simulink model "psk_3"  (Simulink 5.1)
settings: Solver=ode45  StartTime=0.0  StopTime=2  RelTol=1e-3
values from neighbouring files (symbols this model uses):
  fc = 0.2    [TP_fdesign1.m]    (also in TP_fdesign2.m; band4.m = 2000)
  nf = 256    [band4.m]    (also in block_lms_.m = 16)
  Ts = 1/fs    (= 6.25e-05)    [G722_1.m]    (also in adaptiv_2.m = 0.001; adaptiv_3.m = 0.001; adaptiv_4.m = 0.001; adaptiv_5.m = 0.001)
undefined symbols (not defined in the file or in its folder): get, theta
libraries: dspsigops x2, dspmlti3 x2, dspsrcs4 x1, dspsnks4 x1
settings Model: Creator=svenhoffmann  LastModifiedBy=svenhoffmann  ExtModeAutoUpdateStatusClock=off  BooleanDataType=on  ProdHWDeviceType=Microprocessor

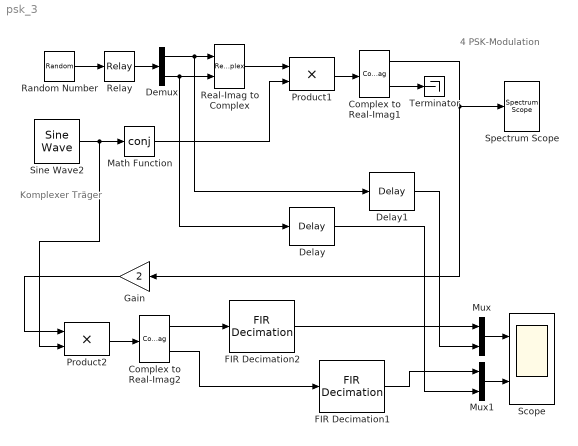
== system psk_3 ==
  note: 4 PSK-Modulation
  note: Komplexer
      | Träger
  Complex to Real-Imag1 : ComplexToRealImag
  Complex to Real-Imag2 : ComplexToRealImag
  Delay : dspsigops/Delay  dly_unit=Samples  delay=nf/2  ic_detail=off  dif_ic_for_ch=off  dif_ic_for_dly=off  ic=0  reset_popup=None
  Delay1 : dspsigops/Delay  dly_unit=Samples  delay=nf/2  ic_detail=off  dif_ic_for_ch=off  dif_ic_for_dly=off  ic=0  reset_popup=None
  Demux : Demux  Outputs=2
  FIR Decimation1 : dspmlti3/FIR Decimation  h=h0  D=10  framing=Maintain input frame size  outputBufInitCond=0  roundingMode=Floor  overflowMode=off
  FIR Decimation2 : dspmlti3/FIR Decimation  h=h0  D=10  framing=Maintain input frame size  outputBufInitCond=0  roundingMode=Floor  overflowMode=off
  Gain : Gain  Orientation=left  Gain=2  SaturateOnIntegerOverflow=on
  Math Function : Math  Operator=conj
  Mux : Mux  Inputs=2
  Mux1 : Mux  Inputs=2
  Product1 : Product  SaturateOnIntegerOverflow=on
  Product2 : Product  SaturateOnIntegerOverflow=on
  Random Number : RandomNumber  Seed=[0124, 769]  SampleTime=100*Ts
  Real-Imag to Complex : RealImagToComplex
  Relay : Relay  OffOutputValue=-1  SampleTime=Ts
  Scope : Scope  NumInputPorts=2
      settings: YMin=-1.5~-1.5  YMax=1.5~1.5
  Sine Wave2 : dspsrcs4/Sine Wave  Amplitude=1  Frequency=fc  Phase=theta  SampleMode=Discrete  OutComplex=Complex  CompMethod=Trigonometric fcn  TableSize=Speed  SampleTime=Ts  SamplesPerFrame=1  dataType=double  wordLen=16  udDataType=sfix(16)  fracBitsMode=Best precision  numFracBits=15  ResetState=Restart at time zero
      settings: additionalParams=on
  Spectrum Scope : dspsnks4/Spectrum Scope  ScopeProperties=off  Domain=Frequency  HorizSpan=1  UseBuffer=on  BufferSize=256  Overlap=64  inpFftLenInherit=off  FFTlength=128  numAvg=10  DisplayProperties=off  AxisGrid=on  Memory=off  FrameNumber=on  AxisLegend=off  AxisZoom=off  OpenScopeAtSimStart=on  OpenScopeImmediately=off  FigPos=get(0,'defaultfigureposition')  AxisProperties=on  XUnits=Hertz  XRange=[0...Fs]  InheritXIncr=off  XIncr=Ts  XLabel=Samples  YUnits=dB  YLabel=Magnitude, dB  LineProperties=off
      settings: YMin=-27.4679460175424  YMax=16.0428342016301
  Terminator : Terminator
  wires:
  Mux/1 -> Scope/1
  Random Number/1 -> Relay/1
  Sine Wave2/1 -> Math Function/1, Product2/2
  Product1/1 -> Complex to Real-Imag1/1
  Complex to Real-Imag1/1 -> Spectrum Scope/1, Gain/1
  Complex to Real-Imag1/2 -> Terminator/1
  Relay/1 -> Demux/1
  Demux/1 -> Real-Imag to Complex/1, Delay1/1
  Demux/2 -> Real-Imag to Complex/2, Delay/1
  Real-Imag to Complex/1 -> Product1/1
  Mux1/1 -> Scope/2
  Delay/1 -> Mux1/2
  Delay1/1 -> Mux/2
  FIR Decimation2/1 -> Mux/1
  FIR Decimation1/1 -> Mux1/1
  Gain/1 -> Product2/1
  Math Function/1 -> Product1/2
  Product2/1 -> Complex to Real-Imag2/1
  Complex to Real-Imag2/1 -> FIR Decimation2/1
  Complex to Real-Imag2/2 -> FIR Decimation1/1
